simulink model "Dion_CBC_Simulink"  (R2023a)
settings: Solver=ode5  StartTime=0.0  StopTime=Inf  FixedStep=0.001  RelTol=1e-3
PostLoadFcn:
  | , if any(exist('dsrtsu_mdlpostloadfcn', 'file') ~= 0), dsrtsu_mdlpostloadfcn('Execute', bdroot); end,
InitFcn:
  | , if any(exist('rtifpga_mdlclblib', 'file') ~= 0), rtifpga_mdlclblib('Init', bdroot); end,
values from neighbouring files (symbols this model uses):
  k_harmonics = 7    [freq_sweep_continous.m]
libraries: simulink x3, rti1202lib_adc_class1 x3, rti1202lib_dac_class1 x1, rti1202lib_base x1
(part 1 of 2)
Description:
  | Standard RTI1202 template.
  | Supported MATLAB version:  R2023a.
settings Model: Tag=RTI1202  DSRTSU_INTERNAL_RTI_VER=620  DSRTSU_INTERNAL_RTI_TYPE=rti1202  RTICANMMDATA=struct('GeneralSetupData',struct('modelroot','C:\Users\VM-User\Desktop\MigrationScripts','generalsettings',struct('filesettings',struct('destfolder',struct('Name','RTICANMM_FILES','Check',1),'buildfolder',struct('Name','.','Check',1),'AbsDestfolder',struct('Name','C:\Users\VM-User\Desktop\MigrationScripts\RTICANMM_FILES'),'AbsBuildfolder',struct('Name','C:\Users\VM-User\Desktop\MigrationScripts'))),'options',struct('addpaths',1,'rmpaths',1,'addtrcexclusion',true,'cannavigator',struct('checkmonitoring',0),'show_usrtrc',0,'use_usrtrc',0),'advanced',struct('options',ones(1,100)),'MPSetup',{{}},'RTI',struct('Type','RTI1202','Ver','7.17','Date','02-Nov-2021'),'modelname','','block','untitled'))  DSRTSU_INTERNAL_RTIFPGA=200  DSRTSU_INTERNAL_RTISTBM_VER=23.1  Creator=akb110  LastModifiedBy=dionl
settings SolverCC: AlgebraicLoopSolver=TrustRegion
settings DataIOCC: ReturnWorkspaceOutputs=off
settings OptimizationCC: BlockReduction=off  OptimizeBlockIOStorage=off  BufferReuse=off  ReuseModelBlockBuffer=off  GlobalBufferReuse=off  ExpressionFolding=off  LocalBlockOutputs=off  OptimizeDataStoreBuffers=off  BusAssignmentInplaceUpdate=off
settings DebuggingCC: UnconnectedInputMsg=warning  UnconnectedOutputMsg=warning  UnconnectedLineMsg=warning  PregeneratedLibrarySubsystemCodeDiagnostic=none  ArithmeticOperatorsInVariantConditions=warning
settings HardwareCC: ProdBitPerPointer=32  ProdBitPerSizeT=32  ProdBitPerPtrDiffT=32  ProdLargestAtomicInteger=Integer  ProdEndianess=BigEndian  ProdWordSize=32  ProdLongLongMode=on  ProdHWDeviceType=Custom Processor->Custom  TargetIntDivRoundTo=Zero  TargetEndianess=BigEndian  TargetHWDeviceType=Custom Processor->Custom
settings ModelReferenceCC: EnableRefExpFcnMdlSchedulingChecks=on  EnableParallelModelReferenceBuilds=on  ParallelModelReferenceMATLABWorkerInit=Load Top Model
settings SFSimCC: SimUseLocalCustomCode=off  MATLABDynamicMemAlloc=off  CustomCodeUndefinedFunction=UseInterfaceOnly
settings RTWCC: Description=dSPACE DS1202 Hardware Platform  SystemTargetFile=rti1202.tlc  MakeCommand=make_rti  TemplateMakefile=rti1202.tmf  RTWUseLocalCustomCode=off  DLArmComputeVersion=19.05
settings CodeAppCC: StateflowObjectComments=on
settings STFCustomTargetCC: TargetLangStandard=C89/C90 (ANSI)  ParMdlRefBuildCompliant=on  ConcurrentExecutionCompliant=off  GRTInterface=off  UseToolchainInfoCompliant=off  SystemTargetFile=rti1202.tlc
settings GRTTargetCC: TargetLangStandard=C89/C90 (ANSI)  CompOptLevelCompliant=off  ConcurrentExecutionCompliant=off  CombineOutputUpdateFcns=off  MatFileLogging=off  CPPClassGenCompliant=off  UseToolchainInfoCompliant=off
settings ConfigComp: CovMetricSettings=dswe

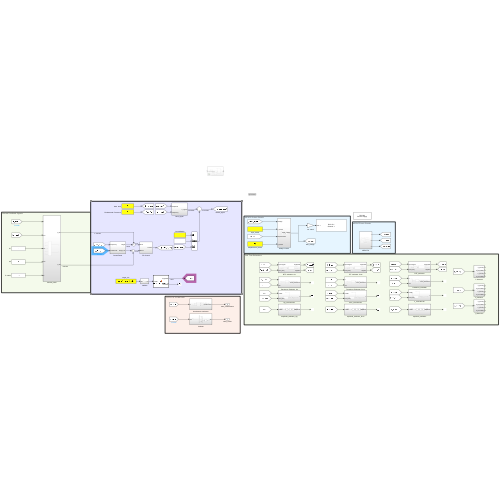
[thumbnail: Simulink's stored preview of the top-level diagram]
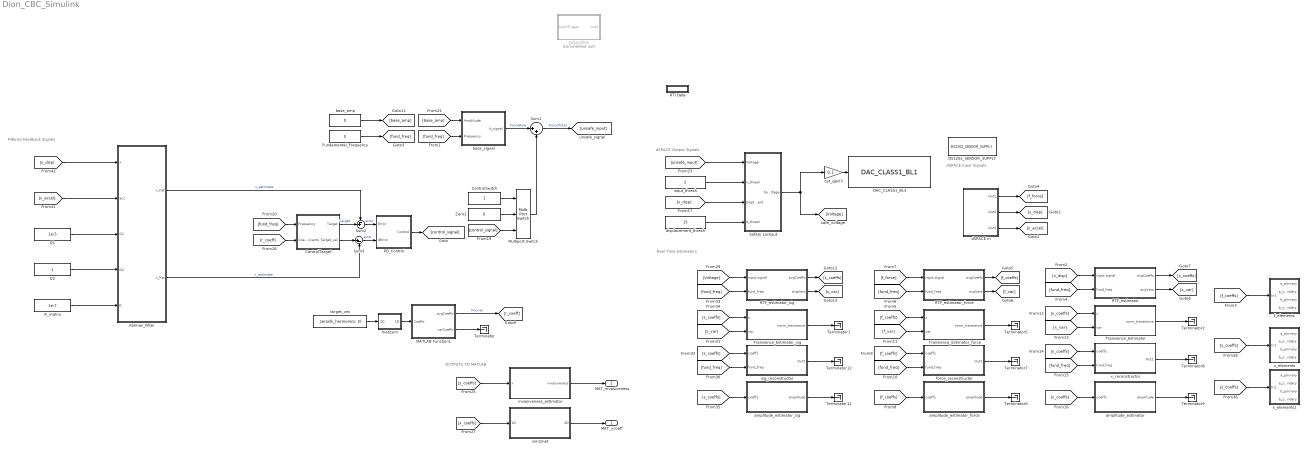
== system Dion_CBC_Simulink ==
  note: OUTPUTS TO MATLAB
  note: Filtered Feedback Signals
  note: Real Time Estimators
  note: dSPACE Input Signals
  note: dSPACE Output Signals
  ControlSwitch : Constant
  ControlTarget : Subsystem
  DAC_CLASS1_BL3 : rti1202lib_dac_class1/DAC_CLASS1_BL1  DSProperties=struct('RTI',struct('Version',uint32(2),'BlockType',struct('isSLSource',uint8(0),'isSLSink',uint8(1),'isHWSource',uint8(0),'isHWSink',uint8(1),'isSetup',uint8(0),'isInline',uint8(1),'isNonInline',uint8(0),'isInterrupt',uint8(0),'isChannelwise',uint8(1)),'IOBoardType',{{'DS120X','STD','DACC1'}},'UnitType','DAC','Identifier','DAC','DialogType','ML','BlockSet','NONE','SlaveProcessor','NONE'))  RTIBlockInterface=struct('InputPortsActive',1,'InputPortsWidth',int32(1),'InputPortsDataType',{{'SS_DOUBLE'}},'InputPortsName',{{['DAC 1']}},'DialogFcn','rti120xstddacc1dacgui','InitLevel',3,'IconTransparency','on','BlockDisplay',{{['DAC CL1\nChannel: 1'],'center'}},'BlockName',struct('Token',{{'DAC_CLASS1_BL1'}}))  RTIBlockParameters=struct('ChannelNo',{{1,'OFF',[]}},'ChannelNumOf',{{1,'OFF',[]}},'InitialValue1',{{0,'OFF',[-10 10]}},'InitialValue2',{{0,'OFF',[-10 10]}},'InitialValue3',{{0,'OFF',[-10 10]}},'InitialValue4',{{0,'OFF',[-10 10]}},'InitialValue5',{{0,'OFF',[-10 10]}},'InitialValue6',{{0,'OFF',[-10 10]}},'InitialValue7',{{0,'OFF',[-10 10]}},'InitialValue8',{{0,'OFF',[-10 10]}},'InitialValue9',{{0,'OFF',[-10 10]}},'InitialValue10',{{0,'OFF',[-10 10]}},'InitialValue11',{{0,'OFF',[-10 10]}},'InitialValue12',{{0,'OFF',[-10 10]}},'InitialValue13',{{0,'OFF',[-10 10]}},'InitialValue14',{{0,'OFF',[-10 10]}},'InitialValue15',{{0,'OFF',[-10 10]}},'InitialValue16',{{0,'OFF',[-10 10]}},'OutputMode',{{ones(1,16),'OFF',[1 2]}},'TermValue1',{{0,'OFF',[-10 10]}},'TermValue2',{{0,'OFF',[-10 10]}},'TermValue3',{{0,'OFF',[-10 10]}},'TermValue4',{{0,'OFF',[-10 10]}},'TermValue5',{{0,'OFF',[-10 10]}},'TermValue6',{{0,'OFF',[-10 10]}},'TermValue7',{{0,'OFF',[-10 10]}},'TermValue8',{{0,'OFF',[-10 10]}},'TermValue9',{{0,'OFF',[-10 10]}},'TermValue10',{{0,'OFF',[-10 10]}},'TermValue11',{{0,'OFF',[-10 10]}},'TermValue12',{{0,'OFF',[-10 10]}},'TermValue13',{{0,'OFF',[-10 10]}},'TermValue14',{{0,'OFF',[-10 10]}},'TermValue15',{{0,'OFF',[-10 10]}},'TermValue16',{{0,'OFF',[-10 10]}},'EnableTermMode',{{0,'OFF',[0 1]}},'TLCFileName',{{'rti120xdac_c1_dac','OFF',[]}},'InitialValueBuildCheck1',{{0,'OFF',[]}},'InitialValueBuildCheck2',{{0,'OFF',[]}},'InitialValueBuildCheck3',{{0,'OFF',[]}},'InitialValueBuildCheck4',{{0,'OFF',[]}},'InitialValueBuildCheck5',{{0,'OFF',[]}},'InitialValueBuildCheck6',{{0,'OFF',[]}},'InitialValueBuildCheck7',{{0,'OFF',[]}},'InitialValueBuildCheck8',{{0,'OFF',[]}},'InitialValueBuildCheck9',{{0,'OFF',[]}},'InitialValueBuildCheck10',{{0,'OFF',[]}},'InitialValueBuildCheck11',{{0,'OFF',[]}},'InitialValueBuildCheck12',{{0,'OFF',[]}},'InitialValueBuildCheck13',{{0,'OFF',[]}},'InitialValueBuildCheck14',{{0,'OFF',[]}},'InitialValueBuildCheck15',{{0,'OFF',[]}},'InitialValueBuildCheck16',{{0,'OFF',[]}},'TermValueBuildCheck1',{{0,'OFF',[]}},'TermValueBuildCheck2',{{0,'OFF',[]}},'TermValueBuildCheck3',{{0,'OFF',[]}},'TermValueBuildCheck4',{{0,'OFF',[]}},'TermValueBuildCheck5',{{0,'OFF',[]}},'TermValueBuildCheck6',{{0,'OFF',[]}},'TermValueBuildCheck7',{{0,'OFF',[]}},'TermValueBuildCheck8',{{0,'OFF',[]}},'TermValueBuildCheck9',{{0,'OFF',[]}},'TermValueBuildCheck10',{{0,'OFF',[]}},'TermValueBuildCheck11',{{0,'OFF',[]}},'TermValueBuildCheck12',{{0,'OFF',[]}},'TermValueBuildCheck13',{{0,'OFF',[]}},'TermValueBuildCheck14',{{0,'OFF',[]}},'TermValueBuildCheck15',{{0,'OFF',[]}},'TermValueBuildCheck16',{{0,'OFF',[]}})  RTISFcnParameters=struct('ChannelNo','int16','ChannelNumOf','int16','InitialValue1','double','InitialValue2','double','InitialValue3','double','InitialValue4','double','InitialValue5','double','InitialValue6','double','InitialValue7','double','InitialValue8','double','InitialValue9','double','InitialValue10','double','InitialValue11','double','InitialValue12','double','InitialValue13','double','InitialValue14','double','InitialValue15','double','InitialValue16','double','OutputMode','int16','TermValue1','double','TermValue2','double','TermValue3','double','TermValue4','double','TermValue5','double','TermValue6','double','TermValue7','double','TermValue8','double','TermValue9','double','TermValue10','double','TermValue11','double','TermValue12','double','TermValue13','double','TermValue14','double','TermValue15','double','TermValue16','double','EnableTermMode','int16','TLCFileName','char')  RTIBlockParaDefault=struct('ChannelNo',1,'ChannelNumOf',1,'InitialValue1',0,'InitialValue2',0,'InitialValue3',0,'InitialValue4',0,'InitialValue5',0,'InitialValue6',0,'InitialValue7',0,'InitialValue8',0,'InitialValue9',0,'InitialValue10',0,'InitialValue11',0,'InitialValue12',0,'InitialValue13',0,'InitialValue14',0,'InitialValue15',0,'InitialValue16',0,'OutputMode',ones(1,16),'TermValue1',0,'TermValue2',0,'TermValue3',0,'TermValue4',0,'TermValue5',0,'TermValue6',0,'TermValue7',0,'TermValue8',0,'TermValue9',0,'TermValue10',0,'TermValue11',0,'TermValue12',0,'TermValue13',0,'TermValue14',0,'TermValue15',0,'TermValue16',0,'EnableTermMode',0,'TLCFileName','rti120xdac_c1_dac','InitialValueBuildCheck1',0,'InitialValueBuildCheck2',0,'InitialValueBuildCheck3',0,'InitialValueBuildCheck4',0,'InitialValueBuildCheck5',0,'InitialValueBuildCheck6',0,'InitialValueBuildCheck7',0,'InitialValueBuildCheck8',0,'InitialValueBuildCheck9',0,'InitialValueBuildCheck10',0,'InitialValueBuildCheck11',0,'InitialValueBuildCheck12',0,'InitialValueBuildCheck13',0,'InitialValueBuildCheck14',0,'InitialValueBuildCheck15',0,'InitialValueBuildCheck16',0,'TermValueBuildCheck1',0,'TermValueBuildCheck2',0,'TermValueBuildCheck3',0,'TermValueBuildCheck4',0,'TermValueBuildCheck5',0,'TermValueBuildCheck6',0,'TermValueBuildCheck7',0,'TermValueBuildCheck8',0,'TermValueBuildCheck9',0,'TermValueBuildCheck10',0,'TermValueBuildCheck11',0,'TermValueBuildCheck12',0,'TermValueBuildCheck13',0,'TermValueBuildCheck14',0,'TermValueBuildCheck15',0,'TermValueBuildCheck16',0)
  DS1202_SENSOR_SUPPLY : rti1202lib_base/DS1202_SENSOR_SUPPLY  DSProperties=struct('RTI',struct('Version',uint32(1),'BlockType',struct('isSLSource',uint8(0),'isSLSink',uint8(0),'isHWSource',uint8(0),'isHWSink',uint8(1),'isSetup',uint8(0),'isInline',uint8(1),'isNonInline',uint8(0),'isInterrupt',uint8(0),'isChannelwise',uint8(0)),'IOBoardType',{{'DS120X','BASE'}},'UnitType','SENSORSUPPLY','Identifier','SENSORSUPPLY','DialogType','ML','BlockSet','NONE','SlaveProcessor','NONE'))  RTIBlockInterface=struct('OutputPortsActive',0,'OutputPortsWidth',int32(0),'DialogFcn','rti120xbasesensorsupplygui','InitLevel',3,'IconTransparency','off','BlockDisplay',{{['DS1202\nSensor Supply'],'center'}},'BlockName',struct('Token',{{'DS1202_SENSOR_SUPPLY'}}))  RTIBlockParameters=struct('Voltage',{{'14','OFF',[2 20]}},'TLCFileName',{{'rti120xbase_sensor_supply','OFF',[]}})  RTISFcnParameters=struct('Voltage','double','TLCFileName','char')  RTIBlockParaDefault=struct('Voltage',2,'TLCFileName','rti120xbase_sensor_supply')
  Fundamental_Frequency : Constant  Value=5
  Kalman_Filter : Subsystem
  MATLAB Function1 : MATLAB Function  TreatAsAtomicUnit=on
  Multiport Switch : MultiPortSwitch  Inputs=2  SaturateOnIntegerOverflow=off  InputSameDT=off
  PD_Control : Subsystem
  Q1 : Constant  Value=1e-5
  Q2 : Constant
  RTF_estimator : Subsystem
  RTF_estimator_force : Subsystem
  RTF_estimator_sig : Subsystem
  RTI Data : Subsystem  Tag=struct('RTIDataServer',struct('RTIDataServerVs','2','RTIModelDescription','struct(''main'',''Dion_CBC_Simulink'',''sub'',''Dion_CBC_Simulink'',''isMp'',0)'))  LoadFcn="if exist('rtidc'), try,  rtidc('DataHostBlockClbLoad', gcbh); catch, disp(['Warning: ''LoadFcn'' for RTI Data block failed: ' lasterr]); end, end,"  mask(RTI_DATA_HOST){}
      mask help:
      | RTI Data Block.
      | This block is used by RTI to store internal model-dependent data.
      | Please keep this block on the root level of the model. Deleting this block will result in data loss.
      |
      | NEVER DELETE OR COPY THIS BLOCK!
      settings: CopyFcn="if exist('rtidc'), try,  rtidc('DataHostBlockClbCopy', gcbh); catch, disp(['Warning: ''CopyFcn'' for RTI Data block failed: ' lasterr]); end, end,"  DeleteFcn="if exist('rtidc'), try,  rtidc('DataHostBlockClbDelete', gcbh); catch, disp(['Warning: ''DeleteFcn'' for RTI Data block failed: ' lasterr]); end, end,"  ModelCloseFcn="if exist('rtidc'), try,  rtidc('DataHostBlockClbModelClose', gcbh); catch, disp(['Warning: ''ModelCloseFcn'' for RTI Data block failed: ' lasterr]); end, end,"  PreSaveFcn="if exist('rtidc'), try,  rtidc('DataHostBlockClbPreSave', gcbh); catch, disp(['Warning: ''PreSaveFcn'' for RTI Data block failed: ' lasterr]); end, end,"  PostSaveFcn="if exist('rtidc'), try,  rtidc('DataHostBlockClbPostSave', gcbh); catch, disp(['Warning: ''PostSaveFcn'' for RTI Data block failed: ' lasterr]); end, end,"  NameChangeFcn="if exist('rtidc'), try,  rtidc('DataHostBlockClbNameChange', gcbh); catch, disp(['Warning: ''NameChangeFcn'' for RTI Data block failed: ' lasterr]); end, end,"
      mask Help:
      | RTI Data Block.
      | This block is used by RTI to store internal model-dependent data.
      | Please keep this block on the root level of the model. Deleting this block will result in data loss.
      | 
      | NEVER DELETE OR COPY THIS BLOCK!
      mask Display:
      | text(0.5, 0.5, 'RTI Data', 'HorizontalAlignment', 'center');
      | plot([1 0]);
  R_matrix : Constant  Value=1e-7
  Safety Lockout : Subsystem
  Subsystem : Subsystem  Commented=on
  Sum1 : Sum  Inputs=|++
  Sum2 : Sum  Inputs=-+|
  Sum3 : Sum  Inputs=|+-
  Terminator{,1..2,5..9,11..12} (10 alike) : Terminator
  Transience_Estimator : Subsystem
  Transience_Estimator_force : Subsystem
  Transience_Estimator_sig : Subsystem
  Zero2 : Constant  Value=0
  amplitude_estimator : Subsystem
  amplitude_estimator_force : Subsystem
  amplitude_estimator_sig : Subsystem
  base_amp : Constant  Value=0
  base_signal : Subsystem
  dSPACE in : Subsystem
  displacement_thresh : Constant  Value=15
  f_elements : Subsystem
  force_reconstructor : Subsystem
  input_thresh : Constant  Value=2
  invasiveness_estimator : Subsystem
  mat2sim : Subsystem
  out_gain3 : Gain  Gain=0.1
  sig_reconstructor : Subsystem
  sim2mat : Subsystem
  target_vec : Constant  Value=zeros(k_harmonics, 2)
  x_elements : Subsystem
  x_elements1 : Subsystem
  x_reconstructor : Subsystem
  MAT_xcoeff : Outport
  MAT_invasiveness : Outport  Port=2
  wires:
  dSPACE in/3(Out3) -> [x_accel]
  [x_disp] -> RTF_estimator/1(input signal)
  [fund_freq] -> RTF_estimator/2(fund_freq)
  Fundamental_Frequency/1 -> [fund_freq]
  amplitude_estimator_force/1(amplitude) -> Terminator6/1
  Transience_Estimator_force/1(norm_transience) -> Terminator5/1
  [fund_freq] -> RTF_estimator_force/2(fund_freq)
  [f_force] -> RTF_estimator_force/1(input signal)
  force_reconstructor/1(Out1) -> Terminator7/1
  RTF_estimator_force/1(avgCoeffs) -> [f_coeffs]
  [f_coeffs] -> Transience_Estimator_force/1(x)
  [f_coeffs] -> amplitude_estimator_force/1(coeffs)
  [f_coeffs] -> force_reconstructor/1(coeffs)
  [fund_freq] -> force_reconstructor/2(fund_freq)
  RTF_estimator_force/2(avgVars) -> [f_var]
  [f_var] -> Transience_Estimator_force/2(var)
  RTF_estimator/1(avgCoeffs) -> [x_coeffs]
  RTF_estimator/2(avgVars) -> [x_var]
  [x_coeffs] -> Transience_Estimator/1(x)
  [x_var] -> Transience_Estimator/2(var)
  Transience_Estimator/1(norm_transience) -> Terminator2/1
  [x_coeffs] -> x_reconstructor/1(coeffs)
  [fund_freq] -> x_reconstructor/2(fund_freq)
  [x_coeffs] -> amplitude_estimator/1(coeffs)
  amplitude_estimator/1(amplitude) -> Terminator9/1
  x_reconstructor/1(Out1) -> Terminator8/1
  [fund_freq] -> base_signal/2(Frequency)
  base_signal/1(b_signal) -> Sum1/1  "ForceRaw"
  Sum1/1 -> [unsafe_input]  "ForceTotal"
  ControlSwitch/1 -> Multiport Switch/1
  Zero2/1 -> Multiport Switch/2
  [control_signal] -> Multiport Switch/3
  Sum2/1 -> PD_Control/1(Error)  "error"
  PD_Control/1(Control) -> [control_signal]
  [fund_freq] -> ControlTarget/1(Frequency)
  Multiport Switch/1 -> Sum1/2
  [x_coeffs] -> sim2mat/1(1D)
  [base_amp] -> base_signal/1(Amplitude)
  [r_coeff] -> ControlTarget/2(Coefficients)
  dSPACE in/2(Out2) -> [x_disp]
  dSPACE in/1(Out1) -> [f_force]
  base_amp/1 -> [base_amp]
  [f_coeffs] -> f_elements/1(In1)
  [x_coeffs] -> x_elements/1(In1)
  [s_coeffs] -> invasiveness_estimator/1(x)
  invasiveness_estimator/1(invasiveness) -> MAT_invasiveness/1
  [s_var] -> Transience_Estimator_sig/2(var)
  RTF_estimator_sig/2(avgVars) -> [s_var]
  [fund_freq] -> sig_reconstructor/2(fund_freq)
  [s_coeffs] -> sig_reconstructor/1(coeffs)
  [s_coeffs] -> amplitude_estimator_sig/1(coeffs)
  [s_coeffs] -> Transience_Estimator_sig/1(x)
  RTF_estimator_sig/1(avgCoeffs) -> [s_coeffs]
  sig_reconstructor/1(Out1) -> Terminator12/1
  [Voltage] -> RTF_estimator_sig/1(input signal)
  [fund_freq] -> RTF_estimator_sig/2(fund_freq)
  Transience_Estimator_sig/1(norm_transience) -> Terminator1/1
  amplitude_estimator_sig/1(amplitude) -> Terminator11/1
  [s_coeffs] -> x_elements1/1(In1)
  Q2/1 -> Kalman_Filter/4(Q2)
  R_matrix/1 -> Kalman_Filter/5(R)
  Kalman_Filter/2(v_hat) -> Sum3/2  "v_estimate"
  Kalman_Filter/1(x_hat) -> Sum2/1  "x_estimate"
  [x_disp] -> Kalman_Filter/1(x)
  [x_accel] -> Kalman_Filter/2(acc)
  Q1/1 -> Kalman_Filter/3(Q1)
  ControlTarget/1(Target) -> Sum2/2  "Target"
  ControlTarget/2(Target_vel) -> Sum3/1
  Sum3/1 -> PD_Control/2(dError)  "error"
  MATLAB Function1/1(avgCoeffs) -> [r_coeff]  "Fourier"
  target_vec/1 -> mat2sim/1(2D)
  MATLAB Function1/2(varCoeffs) -> Terminator/1
  mat2sim/1(1D) -> MATLAB Function1/1(Coeffs)
  sim2mat/1(2D) -> MAT_xcoeff/1
  [unsafe_input] -> Safety Lockout/1(Voltage)
  input_thresh/1 -> Safety Lockout/2(v_thresh)
  [x_disp] -> Safety Lockout/3(Displacement)
  displacement_thresh/1 -> Safety Lockout/4(d_thresh)
  Safety Lockout/1(Safe_Voltage) -> out_gain3/1, [Voltage]
  out_gain3/1 -> DAC_CLASS1_BL3/1

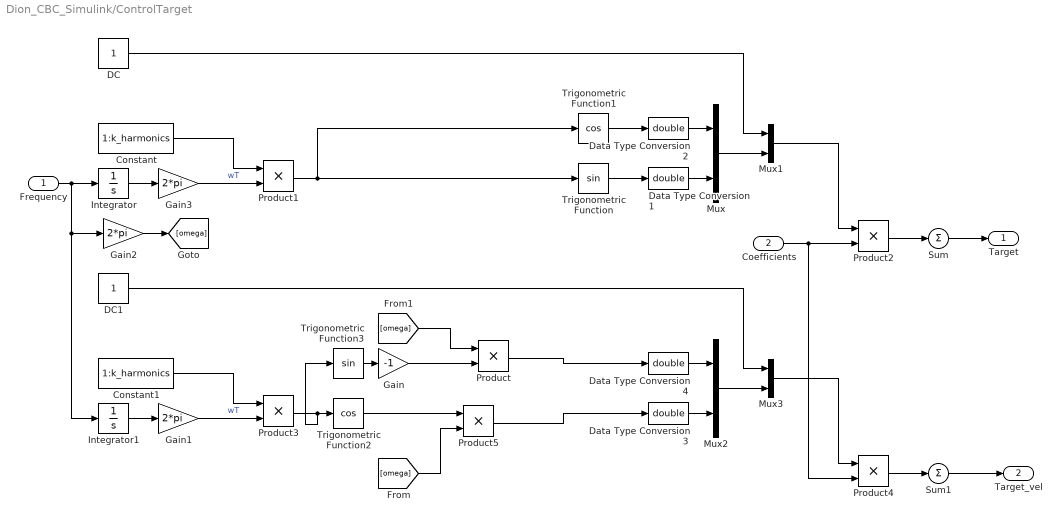
== system Dion_CBC_Simulink/ControlTarget ==
  Frequency : Inport
  Coefficients : Inport  Port=2
  Constant : Constant  Value=1:k_harmonics
  Constant1 : Constant  Value=1:k_harmonics
  DC : Constant
  DC1 : Constant
  Data Type Conversion{1..4} (4 alike) : DataTypeConversion  OutDataTypeStr=double  SaturateOnIntegerOverflow=off  RndMeth=Floor
  Gain : Gain  Gain=-1
  Gain1 : Gain  Gain=2*pi
  Gain2 : Gain  Gain=2*pi
  Gain3 : Gain  Gain=2*pi
  Integrator : Integrator
  Integrator1 : Integrator
  Mux{,1..3} (4 alike) : Mux  Inputs=2
  Product{,1,3,5} (4 alike) : Product
  Product2 : Product  RndMeth=Zero
  Product4 : Product  RndMeth=Zero
  Sum : Sum  Inputs=|+|
  Sum1 : Sum  Inputs=|+|
  Trigonometric Function : Trigonometry
  Trigonometric Function1 : Trigonometry  Operator=cos
  Trigonometric Function2 : Trigonometry  Operator=cos
  Trigonometric Function3 : Trigonometry
  Target : Outport
  Target_vel : Outport  Port=2
  wires:
  Product2/1 -> Sum/1
  Product1/1 -> Trigonometric Function1/1, Trigonometric Function/1
  Sum/1 -> Target/1
  Integrator/1 -> Gain3/1
  Constant/1 -> Product1/1
  Trigonometric Function/1 -> Data Type Conversion1/1
  Mux1/1 -> Product2/1
  Trigonometric Function1/1 -> Data Type Conversion2/1
  Data Type Conversion2/1 -> Mux/1
  Data Type Conversion1/1 -> Mux/2
  Mux/1 -> Mux1/2
  DC/1 -> Mux1/1
  Gain3/1 -> Product1/2  "wT"
  Gain1/1 -> Product3/2  "wT"
  DC1/1 -> Mux3/1
  Mux2/1 -> Mux3/2
  Data Type Conversion3/1 -> Mux2/2
  Data Type Conversion4/1 -> Mux2/1
  Coefficients/1 -> Product4/2, Product2/2
  Trigonometric Function3/1 -> Gain/1
  Mux3/1 -> Product4/1
  Trigonometric Function2/1 -> Product5/1
  Constant1/1 -> Product3/1
  Integrator1/1 -> Gain1/1
  Frequency/1 -> Integrator1/1, Gain2/1, Integrator/1
  Sum1/1 -> Target_vel/1
  Product3/1 -> Trigonometric Function2/1, Trigonometric Function3/1
  Product4/1 -> Sum1/1
  Gain2/1 -> [omega]
  [omega] -> Product/1
  [omega] -> Product5/2
  Product/1 -> Data Type Conversion4/1
  Gain/1 -> Product/2
  Product5/1 -> Data Type Conversion3/1

== system Dion_CBC_Simulink/Kalman_Filter ==
  x : Inport
  acc : Inport  Port=2
  Q1 : Inport  Port=3
  Q2 : Inport  Port=4
  R : Inport  Port=5
  MATLAB Function : MATLAB Function  TreatAsAtomicUnit=on
  x_hat : Outport
  v_hat : Outport  Port=2
  wires:
  R/1 -> MATLAB Function/5(R)
  Q1/1 -> MATLAB Function/3(q1)
  Q2/1 -> MATLAB Function/4(q2)
  acc/1 -> MATLAB Function/2(acc_measured)
  x/1 -> MATLAB Function/1(disp_measured)
  MATLAB Function/1(disp_estimate) -> x_hat/1
  MATLAB Function/2(vel_estimate) -> v_hat/1

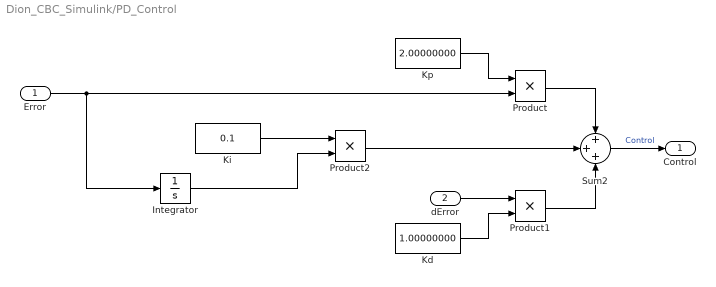
== system Dion_CBC_Simulink/PD_Control ==
  Error : Inport
  dError : Inport  Port=2
  Integrator : Integrator
  Kd : Constant  Value=1.00000000
  Ki : Constant  Value=0.1
  Kp : Constant  Value=2.00000000
  Product : Product  RndMeth=Zero
  Product1 : Product  RndMeth=Zero
  Product2 : Product  RndMeth=Zero
  Sum2 : Sum  Inputs=+++
  Control : Outport
  wires:
  Kp/1 -> Product/1
  Kd/1 -> Product1/2
  Product/1 -> Sum2/1
  Product1/1 -> Sum2/3
  Error/1 -> Integrator/1, Product/2
  Sum2/1 -> Control/1  "Control"
  dError/1 -> Product1/1
  Ki/1 -> Product2/1
  Product2/1 -> Sum2/2
  Integrator/1 -> Product2/2

== system Dion_CBC_Simulink/RTF_estimator ==
  input signal : Inport
  fund_freq : Inport  Port=2
  MATLAB Function1 : MATLAB Function  TreatAsAtomicUnit=on
  Subsystem : Subsystem
  Terminator : Terminator
  avgCoeffs : Outport
  avgVars : Outport  Port=2
  wires:
  input signal/1 -> Subsystem/1(input signal)
  Subsystem/2(Phase1) -> Terminator/1
  fund_freq/1 -> Subsystem/2(fund_freq)
  Subsystem/1(Fourier1) -> MATLAB Function1/1(Coeffs)
  MATLAB Function1/2(varCoeffs) -> avgVars/1
  MATLAB Function1/1(avgCoeffs) -> avgCoeffs/1  "Fourier"

== system Dion_CBC_Simulink/RTF_estimator_force ==
  input signal : Inport
  fund_freq : Inport  Port=2
  MATLAB Function1 : MATLAB Function  TreatAsAtomicUnit=on
  Subsystem : Subsystem
  Terminator : Terminator
  avgCoeffs : Outport
  avgVars : Outport  Port=2
  wires:
  MATLAB Function1/1(avgCoeffs) -> avgCoeffs/1  "Fourier"
  MATLAB Function1/2(varCoeffs) -> avgVars/1
  Subsystem/1(Fourier1) -> MATLAB Function1/1(Coeffs)
  fund_freq/1 -> Subsystem/2(fund_freq)
  Subsystem/2(Phase1) -> Terminator/1
  input signal/1 -> Subsystem/1(input signal)

== system Dion_CBC_Simulink/RTF_estimator_sig ==
  input signal : Inport
  fund_freq : Inport  Port=2
  MATLAB Function1 : MATLAB Function  TreatAsAtomicUnit=on
  Subsystem : Subsystem
  Terminator : Terminator
  avgCoeffs : Outport
  avgVars : Outport  Port=2
  wires:
  input signal/1 -> Subsystem/1(input signal)
  Subsystem/2(Phase1) -> Terminator/1
  fund_freq/1 -> Subsystem/2(fund_freq)
  Subsystem/1(Fourier1) -> MATLAB Function1/1(Coeffs)
  MATLAB Function1/2(varCoeffs) -> avgVars/1
  MATLAB Function1/1(avgCoeffs) -> avgCoeffs/1  "Fourier"

== system Dion_CBC_Simulink/RTI Data ==
  RTI Data Store : Subsystem  Tag="struct('public',struct('sub',struct('name',{{'Dion_CBC_Simulink'}},'data',{{struct('TH',struct('thTaskInfo',struct('taskType',{'TIMER','HWINT','TMRINT','SWINT','GLINT'},'tasksNumOf',{1,0,0,0,0},'srcIds',{{'TIMERA'},{},{},{},{}},'taskNames',{{['Timer Task 1']},{},{},{},{}})),'th_tc',struct('dataType','TASK','taskGroupId','','taskGroupList',{{}},'taskSchedulingPolicy','FCFS','taskType','TIMER','blkh',-1,'srcId','TIMERA','srcSgnName',['Timer A interrupt'],'srcCpuName','','taskName',['Timer Task 1  [0.001] s'],'taskNameDisplayExt','','smplTime',0.001,'smplTimeOffs',0,'hasFixedPriority',0,'priority',1,'hasFixedOvc',0,'ovcType',1,'ovcMax',1),'tc_th',struct('dataType','TASK','taskGroupId','','taskGroupList',{{}},'taskSchedulingPolicy','FCFS','taskType','TIMER','blkh',-1,'srcId','TIMERA','srcSgnName',['Timer A interrupt'],'srcCpuName','','taskName',['Timer Task 1  [0.001] s'],'taskNameDisplayExt','','smplTime',0.001,'smplTimeOffs',0,'hasFixedPriority',0,'priority',1,'hasFixedOvc',0,'ovcType',1,'ovcMax',1))}})),'private',struct('version',struct('dsVer',uint32(2)),'access',struct('modified',['01-Aug-2025 12:46:06'],'type','Model','isPerm',1)))"  mask(RTI_DATA_STORE){}
      mask help:
      | RTI Data Store Block. This block is used by RTI to store internal model dependent data. Deleting this block will result in data loss.
      |
      | NEVER DELETE, COPY, OR MODIFY THIS BLOCK!
      mask Help:
      | RTI Data Store Block. This block is used by RTI to store internal model dependent data. Deleting this block will result in data loss.
      | 
      | NEVER DELETE, COPY, OR MODIFY THIS BLOCK!
      mask Display: text(0.5, 0.5, ' ', 'HorizontalAlignment', 'center');

== system Dion_CBC_Simulink/Safety Lockout ==
  Voltage : Inport
  v_thresh : Inport  Port=2
  Displacement : Inport  Port=3
  d_thresh : Inport  Port=4
  AND : Logic  IconShape=distinctive  AllPortsSameDT=off  OutDataTypeStr=boolean
  No_input1 : Constant  Value=0
  amplitude_switch : Switch  Criteria=u2 > Threshold  SaturateOnIntegerOverflow=off  InputSameDT=off
  input_safety : Subsystem
  output_safety : Subsystem
  Safe_Voltage : Outport
  wires:
  output_safety/1(valid) -> AND/2
  d_thresh/1 -> output_safety/2(threshold)
  input_safety/1(valid) -> AND/1
  amplitude_switch/1 -> Safe_Voltage/1
  No_input1/1 -> amplitude_switch/3
  Voltage/1 -> amplitude_switch/1, input_safety/1(signal)
  v_thresh/1 -> input_safety/2(threshold)
  AND/1 -> amplitude_switch/2
  Displacement/1 -> output_safety/1(signal)

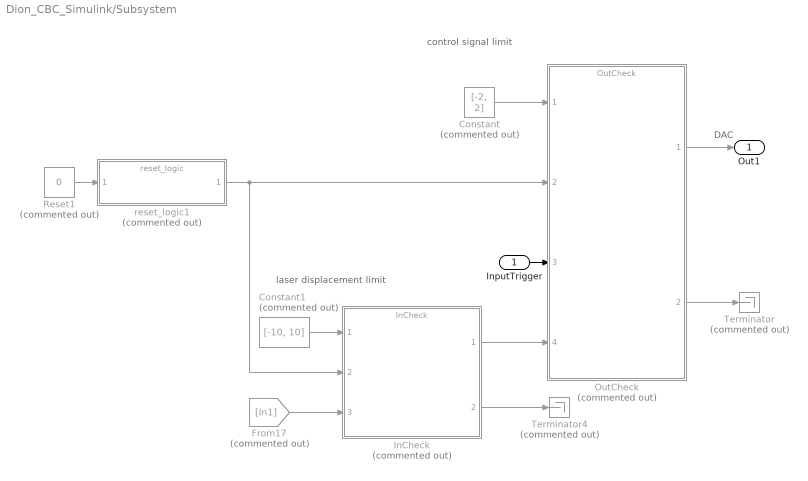
== system Dion_CBC_Simulink/Subsystem ==
  note: DAC
  note: control signal limit
  note: laser displacement limit
  InputTrigger : Inport
  Constant : Constant  Commented=on  Value=[-2, 2]
  Constant1 : Constant  Commented=on  Value=[-10, 10]
  From17 : From  Commented=on  GotoTag=In1
  InCheck : ModelReference  Commented=on  ModelNameDialog=InCheck.slxp  ModelReferenceVersion=1.2  CopyOfModelProtected=on
  OutCheck : ModelReference  Commented=on  ModelNameDialog=OutCheck.slxp  ModelReferenceVersion=1.2  CopyOfModelProtected=on
  Reset1 : Constant  Commented=on  Value=0
  Terminator : Terminator  Commented=on
  Terminator4 : Terminator  Commented=on
  reset_logic1 : ModelReference  Commented=on  ModelNameDialog=reset_logic.slxp  ModelReferenceVersion=1.2  CopyOfModelProtected=on
  Out1 : Outport
  wires:
  InCheck/1 -> OutCheck/4
  InputTrigger/1 -> OutCheck/3
  Reset1/1 -> reset_logic1/1
  OutCheck/2 -> Terminator/1
  reset_logic1/1 -> OutCheck/2, InCheck/2
  From17/1 -> InCheck/3
  InCheck/2 -> Terminator4/1
  OutCheck/1 -> Out1/1
  Constant/1 -> OutCheck/1
  Constant1/1 -> InCheck/1

== system Dion_CBC_Simulink/Transience_Estimator ==
  x : Inport
  var : Inport  Port=2
  Abs1 : Abs  SaturateOnIntegerOverflow=off
  Divide2 : Product  Inputs=*/
  Max : MinMax  Function=max
  get primary1 : Subsystem
  get primary4 : Subsystem
  norm_transience : Outport
  wires:
  Divide2/1 -> Abs1/1
  x/1 -> get primary1/1(Vector)
  get primary1/1(Primary) -> Divide2/2
  get primary4/1(Primary) -> Divide2/1
  var/1 -> get primary4/1(Vector)
  Abs1/1 -> Max/1
  Max/1 -> norm_transience/1

== system Dion_CBC_Simulink/Transience_Estimator_force ==
  x : Inport
  var : Inport  Port=2
  Abs1 : Abs  SaturateOnIntegerOverflow=off
  Divide2 : Product  Inputs=*/
  Max : MinMax  Function=max
  get primary1 : Subsystem
  get primary4 : Subsystem
  norm_transience : Outport
  wires:
  Max/1 -> norm_transience/1
  Abs1/1 -> Max/1
  var/1 -> get primary4/1(Vector)
  get primary4/1(Primary) -> Divide2/1
  get primary1/1(Primary) -> Divide2/2
  x/1 -> get primary1/1(Vector)
  Divide2/1 -> Abs1/1

== system Dion_CBC_Simulink/Transience_Estimator_sig ==
  x : Inport
  var : Inport  Port=2
  Abs1 : Abs  SaturateOnIntegerOverflow=off
  Divide2 : Product  Inputs=*/
  Max : MinMax  Function=max
  get primary1 : Subsystem
  get primary4 : Subsystem
  norm_transience : Outport
  wires:
  Divide2/1 -> Abs1/1
  x/1 -> get primary1/1(Vector)
  get primary1/1(Primary) -> Divide2/2
  get primary4/1(Primary) -> Divide2/1
  var/1 -> get primary4/1(Vector)
  Abs1/1 -> Max/1
  Max/1 -> norm_transience/1

== system Dion_CBC_Simulink/amplitude_estimator ==
  coeffs : Inport
  Sqrt : Sqrt
  Square : Math  Operator=square
  Sum of Elements : Sum  Inputs=+
  amplitude : Outport
  wires:
  Sum of Elements/1 -> Sqrt/1
  Square/1 -> Sum of Elements/1
  coeffs/1 -> Square/1
  Sqrt/1 -> amplitude/1

== system Dion_CBC_Simulink/amplitude_estimator_force ==
  coeffs : Inport
  Sqrt : Sqrt
  Square : Math  Operator=square
  Sum of Elements : Sum  Inputs=+
  amplitude : Outport
  wires:
  Sqrt/1 -> amplitude/1
  coeffs/1 -> Square/1
  Square/1 -> Sum of Elements/1
  Sum of Elements/1 -> Sqrt/1

== system Dion_CBC_Simulink/amplitude_estimator_sig ==
  coeffs : Inport
  Sqrt : Sqrt
  Square : Math  Operator=square
  Sum of Elements : Sum  Inputs=+
  amplitude : Outport
  wires:
  Sum of Elements/1 -> Sqrt/1
  Square/1 -> Sum of Elements/1
  coeffs/1 -> Square/1
  Sqrt/1 -> amplitude/1

== system Dion_CBC_Simulink/base_signal ==
  Amplitude : Inport
  Frequency : Inport  Port=2
  Gain : Gain  Gain=2*pi
  Integrator : Integrator
  Product : Product
  Sin : Trigonometry
  b_signal : Outport
  wires:
  Frequency/1 -> Integrator/1
  Gain/1 -> Sin/1
  Amplitude/1 -> Product/1
  Integrator/1 -> Gain/1
  Sin/1 -> Product/2
  Product/1 -> b_signal/1

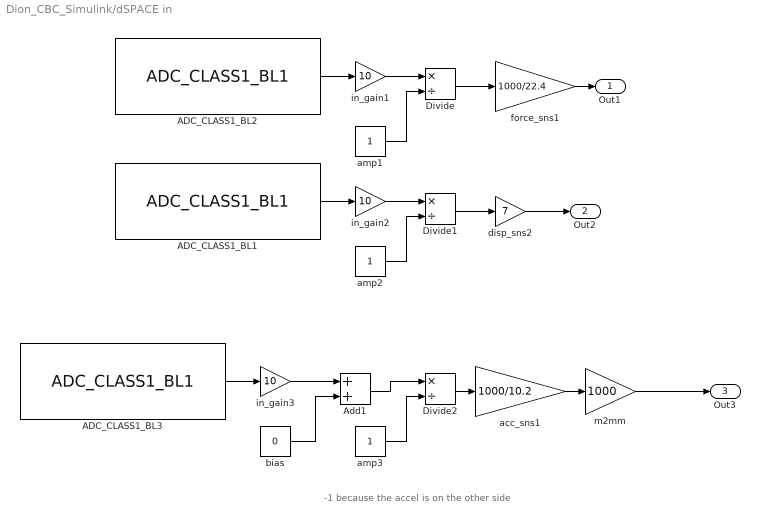
== system Dion_CBC_Simulink/dSPACE in ==
  note: -1 because the accel is on the other side
  ADC_CLASS1_BL1 : rti1202lib_adc_class1/ADC_CLASS1_BL1  DSProperties=struct('RTI',struct('Version',uint32(1),'BlockType',struct('isSLSource',uint8(1),'isSLSink',uint8(1),'isHWSource',uint8(0),'isHWSink',uint8(1),'isSetup',uint8(0),'isInline',uint8(1),'isNonInline',uint8(0),'isInterrupt',uint8(0),'isChannelwise',uint8(1)),'IOBoardType',{{'DS120X','STD','ADCC1'}},'UnitType','ADC','Identifier','ADC','DialogType','ML','BlockSet','NONE','SlaveProcessor','NONE'))  RTIBlockInterface=struct('InputPortsActive',0,'InputPortsWidth',int32(1),'InputPortsDataType',{{'SS_BOOLEAN'}},'InputPortsName',{{'Continue'}},'OutputPortsActive',[1 0],'OutputPortsWidth',int32([1 1]),'OutputPortsDataType',{{'SS_DOUBLE','SS_INT16'}},'OutputPortsName',{{'ADC','Status'}},'DialogFcn','rti120xstdadcc1adcgui','SampleTime',{{-1}},'InitLevel',3,'IconTransparency','on','BlockDisplay',{{['ADC CL1\nChannel: 3'],'center'}},'BlockName',struct('Token',{{'ADC_CLASS1_BL1'}}))  RTIBlockParameters=struct('ReadMode',{{1,'OFF',[1 2]}},'ChannelNo',{{3,'OFF',[]}},'ConversionMode',{{1,'OFF',[1 2]}},'TriggerSource',{{1,'OFF',[1 2]}},'TriggerLineIn',{{1,'OFF',[1 16]}},'SampleMode',{{1,'OFF',[1 2]}},'BurstTriggerSource',{{1,'OFF',[1 2]}},'BurstTriggerLine',{{1,'OFF',[1 16]}},'ConvTriggerSource',{{3,'OFF',[1 3]}},'ConvTriggerLine',{{1,'OFF',[1 16]}},'ConvPeriod',{{'100e-6','OFF',[1e-6 1.34]}},'ConvPeriodCheck',{{0,'OFF',[]}},'BurstSize',{{'10','OFF',[]}},'BurstSizeCheck',{{0,'OFF',[]}},'DataSetOffset',{{'0','OFF',[]}},'DataSetOffsetCheck',{{0,'OFF',[]}},'DataSetLength',{{'1','OFF',[]}},'DataSetLengthCheck',{{0,'OFF',[]}},'EnableTriggerEvent',{{0,'OFF',[0 1]}},'TriggerMode',{{2,'OFF',[1 3]}},'TriggerLineOut',{{1,'OFF',[1 16]}},'ADCSWStartEnable',{{0,'OFF',[0 1]}},'SampleTime',{{'-1','OFF',[-1 inf]}},'SampleTimeCheck',{{1,'OFF',[]}},'StatusPortEnable',{{0,'OFF',[0 1]}},'TLCFileName',{{'rti120xadc_c1_adc','OFF',[]}})  RTISFcnParameters=struct('ReadMode','int16','ChannelNo','int16','ConversionMode','int16','TriggerSource','int16','TriggerLineIn','int16','SampleMode','int16','BurstTriggerSource','int16','BurstTriggerLine','int16','ConvTriggerSource','int16','ConvTriggerLine','int16','ConvPeriod','double','BurstSize','int16','DataSetOffset','int16','DataSetLength','int16','EnableTriggerEvent','int16','TriggerMode','int16','TriggerLineOut','int16','ADCSWStartEnable','int16','SampleTime','double','StatusPortEnable','int16','TLCFileName','char')  RTIBlockParaDefault=struct('ReadMode',1,'ChannelNo',1,'ConversionMode',1,'TriggerSource',1,'TriggerLineIn',1,'SampleMode',1,'BurstTriggerSource',1,'BurstTriggerLine',1,'ConvTriggerSource',3,'ConvTriggerLine',1,'ConvPeriod',0.0001,'ConvPeriodCheck',0,'BurstSize',10,'BurstSizeCheck',0,'DataSetOffset',0,'DataSetOffsetCheck',0,'DataSetLength',1,'DataSetLengthCheck',0,'EnableTriggerEvent',0,'TriggerMode',2,'TriggerLineOut',1,'ADCSWStartEnable',0,'SampleTime',-1,'SampleTimeCheck',1,'StatusPortEnable',0,'TLCFileName','rti120xadc_c1_adc')
  ADC_CLASS1_BL2 : rti1202lib_adc_class1/ADC_CLASS1_BL1  DSProperties=struct('RTI',struct('Version',uint32(1),'BlockType',struct('isSLSource',uint8(1),'isSLSink',uint8(1),'isHWSource',uint8(0),'isHWSink',uint8(1),'isSetup',uint8(0),'isInline',uint8(1),'isNonInline',uint8(0),'isInterrupt',uint8(0),'isChannelwise',uint8(1)),'IOBoardType',{{'DS120X','STD','ADCC1'}},'UnitType','ADC','Identifier','ADC','DialogType','ML','BlockSet','NONE','SlaveProcessor','NONE'))  RTIBlockInterface=struct('InputPortsActive',0,'InputPortsWidth',int32(1),'InputPortsDataType',{{'SS_BOOLEAN'}},'InputPortsName',{{'Continue'}},'OutputPortsActive',[1 0],'OutputPortsWidth',int32([1 1]),'OutputPortsDataType',{{'SS_DOUBLE','SS_INT16'}},'OutputPortsName',{{'ADC','Status'}},'DialogFcn','rti120xstdadcc1adcgui','SampleTime',{{-1}},'InitLevel',3,'IconTransparency','on','BlockDisplay',{{['ADC CL1\nChannel: 1'],'center'}},'BlockName',struct('Token',{{'ADC_CLASS1_BL1'}}))  RTIBlockParameters=struct('ReadMode',{{1,'OFF',[1 2]}},'ChannelNo',{{1,'OFF',[]}},'ConversionMode',{{1,'OFF',[1 2]}},'TriggerSource',{{1,'OFF',[1 2]}},'TriggerLineIn',{{1,'OFF',[1 16]}},'SampleMode',{{1,'OFF',[1 2]}},'BurstTriggerSource',{{1,'OFF',[1 2]}},'BurstTriggerLine',{{1,'OFF',[1 16]}},'ConvTriggerSource',{{3,'OFF',[1 3]}},'ConvTriggerLine',{{1,'OFF',[1 16]}},'ConvPeriod',{{'100e-6','OFF',[1e-6 1.34]}},'ConvPeriodCheck',{{0,'OFF',[]}},'BurstSize',{{'10','OFF',[]}},'BurstSizeCheck',{{0,'OFF',[]}},'DataSetOffset',{{'0','OFF',[]}},'DataSetOffsetCheck',{{0,'OFF',[]}},'DataSetLength',{{'1','OFF',[]}},'DataSetLengthCheck',{{0,'OFF',[]}},'EnableTriggerEvent',{{0,'OFF',[0 1]}},'TriggerMode',{{2,'OFF',[1 3]}},'TriggerLineOut',{{1,'OFF',[1 16]}},'ADCSWStartEnable',{{0,'OFF',[0 1]}},'SampleTime',{{'-1','OFF',[-1 inf]}},'SampleTimeCheck',{{1,'OFF',[]}},'StatusPortEnable',{{0,'OFF',[0 1]}},'TLCFileName',{{'rti120xadc_c1_adc','OFF',[]}})  RTISFcnParameters=struct('ReadMode','int16','ChannelNo','int16','ConversionMode','int16','TriggerSource','int16','TriggerLineIn','int16','SampleMode','int16','BurstTriggerSource','int16','BurstTriggerLine','int16','ConvTriggerSource','int16','ConvTriggerLine','int16','ConvPeriod','double','BurstSize','int16','DataSetOffset','int16','DataSetLength','int16','EnableTriggerEvent','int16','TriggerMode','int16','TriggerLineOut','int16','ADCSWStartEnable','int16','SampleTime','double','StatusPortEnable','int16','TLCFileName','char')  RTIBlockParaDefault=struct('ReadMode',1,'ChannelNo',1,'ConversionMode',1,'TriggerSource',1,'TriggerLineIn',1,'SampleMode',1,'BurstTriggerSource',1,'BurstTriggerLine',1,'ConvTriggerSource',3,'ConvTriggerLine',1,'ConvPeriod',0.0001,'ConvPeriodCheck',0,'BurstSize',10,'BurstSizeCheck',0,'DataSetOffset',0,'DataSetOffsetCheck',0,'DataSetLength',1,'DataSetLengthCheck',0,'EnableTriggerEvent',0,'TriggerMode',2,'TriggerLineOut',1,'ADCSWStartEnable',0,'SampleTime',-1,'SampleTimeCheck',1,'StatusPortEnable',0,'TLCFileName','rti120xadc_c1_adc')
  ADC_CLASS1_BL3 : rti1202lib_adc_class1/ADC_CLASS1_BL1  DSProperties=struct('RTI',struct('Version',uint32(1),'BlockType',struct('isSLSource',uint8(1),'isSLSink',uint8(1),'isHWSource',uint8(0),'isHWSink',uint8(1),'isSetup',uint8(0),'isInline',uint8(1),'isNonInline',uint8(0),'isInterrupt',uint8(0),'isChannelwise',uint8(1)),'IOBoardType',{{'DS120X','STD','ADCC1'}},'UnitType','ADC','Identifier','ADC','DialogType','ML','BlockSet','NONE','SlaveProcessor','NONE'))  RTIBlockInterface=struct('InputPortsActive',0,'InputPortsWidth',int32(1),'InputPortsDataType',{{'SS_BOOLEAN'}},'InputPortsName',{{'Continue'}},'OutputPortsActive',[1 0],'OutputPortsWidth',int32([1 1]),'OutputPortsDataType',{{'SS_DOUBLE','SS_INT16'}},'OutputPortsName',{{'ADC','Status'}},'DialogFcn','rti120xstdadcc1adcgui','SampleTime',{{-1}},'InitLevel',3,'IconTransparency','on','BlockDisplay',{{['ADC CL1\nChannel: 2'],'center'}},'BlockName',struct('Token',{{'ADC_CLASS1_BL1'}}))  RTIBlockParameters=struct('ReadMode',{{1,'OFF',[1 2]}},'ChannelNo',{{2,'OFF',[]}},'ConversionMode',{{1,'OFF',[1 2]}},'TriggerSource',{{1,'OFF',[1 2]}},'TriggerLineIn',{{1,'OFF',[1 16]}},'SampleMode',{{1,'OFF',[1 2]}},'BurstTriggerSource',{{1,'OFF',[1 2]}},'BurstTriggerLine',{{1,'OFF',[1 16]}},'ConvTriggerSource',{{3,'OFF',[1 3]}},'ConvTriggerLine',{{1,'OFF',[1 16]}},'ConvPeriod',{{'100e-6','OFF',[1e-6 1.34]}},'ConvPeriodCheck',{{0,'OFF',[]}},'BurstSize',{{'10','OFF',[]}},'BurstSizeCheck',{{0,'OFF',[]}},'DataSetOffset',{{'0','OFF',[]}},'DataSetOffsetCheck',{{0,'OFF',[]}},'DataSetLength',{{'1','OFF',[]}},'DataSetLengthCheck',{{0,'OFF',[]}},'EnableTriggerEvent',{{0,'OFF',[0 1]}},'TriggerMode',{{2,'OFF',[1 3]}},'TriggerLineOut',{{1,'OFF',[1 16]}},'ADCSWStartEnable',{{0,'OFF',[0 1]}},'SampleTime',{{'-1','OFF',[-1 inf]}},'SampleTimeCheck',{{1,'OFF',[]}},'StatusPortEnable',{{0,'OFF',[0 1]}},'TLCFileName',{{'rti120xadc_c1_adc','OFF',[]}})  RTISFcnParameters=struct('ReadMode','int16','ChannelNo','int16','ConversionMode','int16','TriggerSource','int16','TriggerLineIn','int16','SampleMode','int16','BurstTriggerSource','int16','BurstTriggerLine','int16','ConvTriggerSource','int16','ConvTriggerLine','int16','ConvPeriod','double','BurstSize','int16','DataSetOffset','int16','DataSetLength','int16','EnableTriggerEvent','int16','TriggerMode','int16','TriggerLineOut','int16','ADCSWStartEnable','int16','SampleTime','double','StatusPortEnable','int16','TLCFileName','char')  RTIBlockParaDefault=struct('ReadMode',1,'ChannelNo',1,'ConversionMode',1,'TriggerSource',1,'TriggerLineIn',1,'SampleMode',1,'BurstTriggerSource',1,'BurstTriggerLine',1,'ConvTriggerSource',3,'ConvTriggerLine',1,'ConvPeriod',0.0001,'ConvPeriodCheck',0,'BurstSize',10,'BurstSizeCheck',0,'DataSetOffset',0,'DataSetOffsetCheck',0,'DataSetLength',1,'DataSetLengthCheck',0,'EnableTriggerEvent',0,'TriggerMode',2,'TriggerLineOut',1,'ADCSWStartEnable',0,'SampleTime',-1,'SampleTimeCheck',1,'StatusPortEnable',0,'TLCFileName','rti120xadc_c1_adc')
  Add1 : Sum
  Divide : Product  Inputs=*/
  Divide1 : Product  Inputs=*/
  Divide2 : Product  Inputs=*/
  acc_sns1 : Gain  Gain=1000/10.2
  amp1 : Constant
  amp2 : Constant
  amp3 : Constant
  bias : Constant  Value=0
  disp_sns2 : Gain  Gain=7
  force_sns1 : Gain  Gain=1000/22.4
  in_gain1 : Gain  Gain=10
  in_gain2 : Gain  Gain=10
  in_gain3 : Gain  Gain=10
  m2mm : Gain  Gain=1000
  Out1 : Outport
  Out2 : Outport  Port=2
  Out3 : Outport  Port=3
  wires:
  ADC_CLASS1_BL2/1 -> in_gain1/1
  Divide1/1 -> disp_sns2/1
  amp2/1 -> Divide1/2
  ADC_CLASS1_BL1/1 -> in_gain2/1
  in_gain2/1 -> Divide1/1
  in_gain1/1 -> Divide/1
  Divide/1 -> force_sns1/1
  amp1/1 -> Divide/2
  force_sns1/1 -> Out1/1
  acc_sns1/1 -> m2mm/1
  amp3/1 -> Divide2/2
  ADC_CLASS1_BL3/1 -> in_gain3/1
  Divide2/1 -> acc_sns1/1
  disp_sns2/1 -> Out2/1
  m2mm/1 -> Out3/1
  in_gain3/1 -> Add1/1
  Add1/1 -> Divide2/1
  bias/1 -> Add1/2

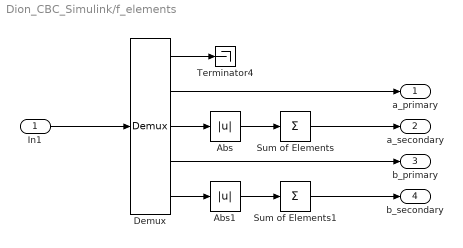
== system Dion_CBC_Simulink/f_elements ==
  In1 : Inport
  Abs : Abs  SaturateOnIntegerOverflow=off
  Abs1 : Abs  SaturateOnIntegerOverflow=off
  Demux : Demux  Outputs=[1, 1, k_harmonics-1, 1, k_harmonics-1]
  Sum of Elements : Sum  Inputs=+
  Sum of Elements1 : Sum  Inputs=+
  Terminator4 : Terminator
  a_primary : Outport
  a_secondary : Outport  Port=2
  b_primary : Outport  Port=3
  b_secondary : Outport  Port=4
  wires:
  Abs/1 -> Sum of Elements/1
  Demux/3 -> Abs/1
  Demux/1 -> Terminator4/1
  Demux/2 -> a_primary/1
  Demux/5 -> Abs1/1
  In1/1 -> Demux/1
  Abs1/1 -> Sum of Elements1/1
  Sum of Elements/1 -> a_secondary/1
  Sum of Elements1/1 -> b_secondary/1
  Demux/4 -> b_primary/1

== system Dion_CBC_Simulink/force_reconstructor ==
  coeffs : Inport
  fund_freq : Inport  Port=2
  Harmonic Basis Gen1 : Subsystem
  Product : Product
  Sum of Elements : Sum  Inputs=+
  Out1 : Outport
  wires:
  Product/1 -> Sum of Elements/1
  fund_freq/1 -> Harmonic Basis Gen1/1(fund_freq)
  Harmonic Basis Gen1/1(harmonic_basis) -> Product/2
  coeffs/1 -> Product/1
  Sum of Elements/1 -> Out1/1

== system Dion_CBC_Simulink/invasiveness_estimator ==
  x : Inport
  Abs1 : Abs  SaturateOnIntegerOverflow=off
  Abs2 : Abs  SaturateOnIntegerOverflow=off
  Divide1 : Product  Inputs=*/
  Sum of Elements : Sum  Inputs=+
  Sum of Elements1 : Sum  Inputs=+
  get primary1 : Subsystem
  get secondary : Subsystem
  invasiveness : Outport
  wires:
  get secondary/1(secondary) -> Abs1/1
  x/1 -> get secondary/1(Vector), get primary1/1(Vector)
  get primary1/1(Primary) -> Abs2/1
  Abs1/1 -> Sum of Elements/1
  Abs2/1 -> Sum of Elements1/1
  Sum of Elements/1 -> Divide1/1
  Sum of Elements1/1 -> Divide1/2
  Divide1/1 -> invasiveness/1

== system Dion_CBC_Simulink/mat2sim ==
  2D : Inport
  DC : Constant  Value=0
  Mux : Mux  Inputs=2
  Reshape : Reshape  OutputDimensionality=Customize  OutputDimensions=[2*k_harmonics,1]
  1D : Outport
  wires:
  2D/1 -> Reshape/1
  DC/1 -> Mux/1
  Mux/1 -> 1D/1
  Reshape/1 -> Mux/2

== system Dion_CBC_Simulink/sig_reconstructor ==
  coeffs : Inport
  fund_freq : Inport  Port=2
  Harmonic Basis Gen1 : Subsystem
  Product : Product
  Sum of Elements : Sum  Inputs=+
  Out1 : Outport
  wires:
  Sum of Elements/1 -> Out1/1
  coeffs/1 -> Product/1
  Harmonic Basis Gen1/1(harmonic_basis) -> Product/2
  fund_freq/1 -> Harmonic Basis Gen1/1(fund_freq)
  Product/1 -> Sum of Elements/1

== system Dion_CBC_Simulink/sim2mat ==
  1D : Inport
  Demux1 : Demux  Outputs=[1, k_harmonics, k_harmonics]
  Mux : Mux  Inputs=2
  Reshape : Reshape  OutputDimensionality=Customize  OutputDimensions=[k_harmonics,2]
  Terminator : Terminator
  2D : Outport
  wires:
  Mux/1 -> Reshape/1
  Reshape/1 -> 2D/1
  Demux1/3 -> Mux/2
  Demux1/2 -> Mux/1
  Demux1/1 -> Terminator/1
  1D/1 -> Demux1/1

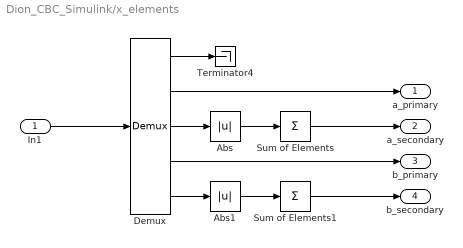
== system Dion_CBC_Simulink/x_elements ==
  In1 : Inport
  Abs : Abs  SaturateOnIntegerOverflow=off
  Abs1 : Abs  SaturateOnIntegerOverflow=off
  Demux : Demux  Outputs=[1, 1, k_harmonics-1, 1, k_harmonics-1]
  Sum of Elements : Sum  Inputs=+
  Sum of Elements1 : Sum  Inputs=+
  Terminator4 : Terminator
  a_primary : Outport
  a_secondary : Outport  Port=2
  b_primary : Outport  Port=3
  b_secondary : Outport  Port=4
  wires:
  Demux/4 -> b_primary/1
  Sum of Elements1/1 -> b_secondary/1
  Sum of Elements/1 -> a_secondary/1
  Abs1/1 -> Sum of Elements1/1
  In1/1 -> Demux/1
  Demux/5 -> Abs1/1
  Demux/2 -> a_primary/1
  Demux/1 -> Terminator4/1
  Demux/3 -> Abs/1
  Abs/1 -> Sum of Elements/1

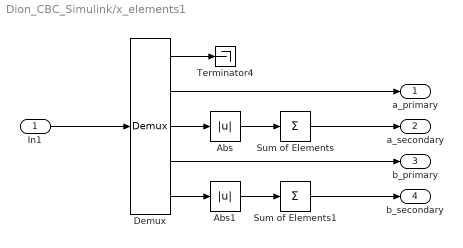
== system Dion_CBC_Simulink/x_elements1 ==
  In1 : Inport
  Abs : Abs  SaturateOnIntegerOverflow=off
  Abs1 : Abs  SaturateOnIntegerOverflow=off
  Demux : Demux  Outputs=[1, 1, k_harmonics-1, 1, k_harmonics-1]
  Sum of Elements : Sum  Inputs=+
  Sum of Elements1 : Sum  Inputs=+
  Terminator4 : Terminator
  a_primary : Outport
  a_secondary : Outport  Port=2
  b_primary : Outport  Port=3
  b_secondary : Outport  Port=4
  wires:
  Abs/1 -> Sum of Elements/1
  Demux/3 -> Abs/1
  Demux/1 -> Terminator4/1
  Demux/2 -> a_primary/1
  Demux/5 -> Abs1/1
  In1/1 -> Demux/1
  Abs1/1 -> Sum of Elements1/1
  Sum of Elements/1 -> a_secondary/1
  Sum of Elements1/1 -> b_secondary/1
  Demux/4 -> b_primary/1

== system Dion_CBC_Simulink/x_reconstructor ==
  coeffs : Inport
  fund_freq : Inport  Port=2
  Harmonic Basis Gen1 : Subsystem
  Product : Product
  Sum of Elements : Sum  Inputs=+
  Out1 : Outport
  wires:
  Sum of Elements/1 -> Out1/1
  coeffs/1 -> Product/1
  Harmonic Basis Gen1/1(harmonic_basis) -> Product/2
  fund_freq/1 -> Harmonic Basis Gen1/1(fund_freq)
  Product/1 -> Sum of Elements/1

== system Dion_CBC_Simulink/RTF_estimator/Subsystem ==
  input signal : Inport
  fund_freq : Inport  Port=2
  Fourier Series 2 : Subsystem
  Harmonic Basis Gen1 : Subsystem
  Fourier1 : Outport
  Phase1 : Outport  Port=2
  wires:
  Fourier Series 2/2(Phase) -> Phase1/1
  input signal/1 -> Fourier Series 2/1(input signal)
  Fourier Series 2/1(Fourier) -> Fourier1/1
  fund_freq/1 -> Harmonic Basis Gen1/1(fund_freq), Fourier Series 2/3(fundamental frequency)
  Harmonic Basis Gen1/1(harmonic_basis) -> Fourier Series 2/2(harmonic basis)

== system Dion_CBC_Simulink/RTF_estimator_force/Subsystem ==
  input signal : Inport
  fund_freq : Inport  Port=2
  Fourier Series 2 : Subsystem
  Harmonic Basis Gen1 : Subsystem
  Fourier1 : Outport
  Phase1 : Outport  Port=2
  wires:
  Harmonic Basis Gen1/1(harmonic_basis) -> Fourier Series 2/2(harmonic basis)
  fund_freq/1 -> Fourier Series 2/3(fundamental frequency), Harmonic Basis Gen1/1(fund_freq)
  Fourier Series 2/1(Fourier) -> Fourier1/1
  input signal/1 -> Fourier Series 2/1(input signal)
  Fourier Series 2/2(Phase) -> Phase1/1

== system Dion_CBC_Simulink/RTF_estimator_sig/Subsystem ==
  input signal : Inport
  fund_freq : Inport  Port=2
  Fourier Series 2 : Subsystem
  Harmonic Basis Gen1 : Subsystem
  Fourier1 : Outport
  Phase1 : Outport  Port=2
  wires:
  Fourier Series 2/2(Phase) -> Phase1/1
  input signal/1 -> Fourier Series 2/1(input signal)
  Fourier Series 2/1(Fourier) -> Fourier1/1
  fund_freq/1 -> Harmonic Basis Gen1/1(fund_freq), Fourier Series 2/3(fundamental frequency)
  Harmonic Basis Gen1/1(harmonic_basis) -> Fourier Series 2/2(harmonic basis)

== system Dion_CBC_Simulink/RTI Data/RTI Data Store ==
  RTI Data Store : Subsystem  mask(RTI_DATA_STORE){}
      mask help:
      | RTI Data Store Block. This block is used by RTI to store internal model dependent data. Deleting this block will result in data loss.
      |
      | NEVER DELETE, COPY, OR MODIFY THIS BLOCK!
      mask Help:
      | RTI Data Store Block. This block is used by RTI to store internal model dependent data. Deleting this block will result in data loss.
      | 
      | NEVER DELETE, COPY, OR MODIFY THIS BLOCK!
      mask Display: text(0.5, 0.5, ' ', 'HorizontalAlignment', 'center');

== system Dion_CBC_Simulink/Safety Lockout/input_safety ==
  signal : Inport
  threshold : Inport  Port=2
  Abs : Abs  SaturateOnIntegerOverflow=off
  Less Than : RelationalOperator  Operator=<  OutDataTypeStr=boolean  RndMeth=Simplest  InputSameDT=off
  valid : Outport
  wires:
  Abs/1 -> Less Than/1
  signal/1 -> Abs/1
  threshold/1 -> Less Than/2
  Less Than/1 -> valid/1

== system Dion_CBC_Simulink/Safety Lockout/output_safety ==
  signal : Inport
  threshold : Inport  Port=2
  Abs : Abs  SaturateOnIntegerOverflow=off
  Less Than : RelationalOperator  Operator=<  OutDataTypeStr=boolean  RndMeth=Simplest  InputSameDT=off
  valid : Outport
  wires:
  Less Than/1 -> valid/1
  threshold/1 -> Less Than/2
  signal/1 -> Abs/1
  Abs/1 -> Less Than/1

== system Dion_CBC_Simulink/Transience_Estimator/get primary1 ==
  Vector : Inport
  Demux : Demux  Outputs=[1, 1, k_harmonics-1, 1, k_harmonics-1]
  Mux : Mux  Inputs=2
  Terminator2 : Terminator
  Terminator3 : Terminator
  Terminator4 : Terminator
  Primary : Outport
  wires:
  Vector/1 -> Demux/1
  Demux/5 -> Terminator4/1
  Demux/3 -> Terminator3/1
  Mux/1 -> Primary/1
  Demux/4 -> Mux/2
  Demux/2 -> Mux/1
  Demux/1 -> Terminator2/1

== system Dion_CBC_Simulink/Transience_Estimator/get primary4 ==
  Vector : Inport
  Demux : Demux  Outputs=[1, 1, k_harmonics-1, 1, k_harmonics-1]
  Mux : Mux  Inputs=2
  Terminator2 : Terminator
  Terminator3 : Terminator
  Terminator4 : Terminator
  Primary : Outport
  wires:
  Demux/1 -> Terminator2/1
  Demux/2 -> Mux/1
  Demux/4 -> Mux/2
  Mux/1 -> Primary/1
  Demux/3 -> Terminator3/1
  Demux/5 -> Terminator4/1
  Vector/1 -> Demux/1

== system Dion_CBC_Simulink/Transience_Estimator_force/get primary1 ==
  Vector : Inport
  Demux : Demux  Outputs=[1, 1, k_harmonics-1, 1, k_harmonics-1]
  Mux : Mux  Inputs=2
  Terminator2 : Terminator
  Terminator3 : Terminator
  Terminator4 : Terminator
  Primary : Outport
  wires:
  Demux/1 -> Terminator2/1
  Demux/2 -> Mux/1
  Demux/4 -> Mux/2
  Mux/1 -> Primary/1
  Demux/3 -> Terminator3/1
  Demux/5 -> Terminator4/1
  Vector/1 -> Demux/1

== system Dion_CBC_Simulink/Transience_Estimator_force/get primary4 ==
  Vector : Inport
  Demux : Demux  Outputs=[1, 1, k_harmonics-1, 1, k_harmonics-1]
  Mux : Mux  Inputs=2
  Terminator2 : Terminator
  Terminator3 : Terminator
  Terminator4 : Terminator
  Primary : Outport
  wires:
  Vector/1 -> Demux/1
  Demux/5 -> Terminator4/1
  Demux/3 -> Terminator3/1
  Mux/1 -> Primary/1
  Demux/4 -> Mux/2
  Demux/2 -> Mux/1
  Demux/1 -> Terminator2/1

== system Dion_CBC_Simulink/Transience_Estimator_sig/get primary1 ==
  Vector : Inport
  Demux : Demux  Outputs=[1, 1, k_harmonics-1, 1, k_harmonics-1]
  Mux : Mux  Inputs=2
  Terminator2 : Terminator
  Terminator3 : Terminator
  Terminator4 : Terminator
  Primary : Outport
  wires:
  Vector/1 -> Demux/1
  Demux/5 -> Terminator4/1
  Demux/3 -> Terminator3/1
  Mux/1 -> Primary/1
  Demux/4 -> Mux/2
  Demux/2 -> Mux/1
  Demux/1 -> Terminator2/1

== system Dion_CBC_Simulink/Transience_Estimator_sig/get primary4 ==
  Vector : Inport
  Demux : Demux  Outputs=[1, 1, k_harmonics-1, 1, k_harmonics-1]
  Mux : Mux  Inputs=2
  Terminator2 : Terminator
  Terminator3 : Terminator
  Terminator4 : Terminator
  Primary : Outport
  wires:
  Demux/1 -> Terminator2/1
  Demux/2 -> Mux/1
  Demux/4 -> Mux/2
  Mux/1 -> Primary/1
  Demux/3 -> Terminator3/1
  Demux/5 -> Terminator4/1
  Vector/1 -> Demux/1

== system Dion_CBC_Simulink/force_reconstructor/Harmonic Basis Gen1 ==
  fund_freq : Inport
  Cos : Trigonometry  Operator=cos
  DC : Constant
  Gain1 : Gain  Gain=2*pi
  Integrator : Integrator
  Mux : Mux  Inputs=3
  Product : Product
  Sin : Trigonometry
  harmonics_array : Constant  Value=1:k_harmonics
  harmonic_basis : Outport  OutDataTypeStr=double  SampleTime=0
  wires:
  DC/1 -> Mux/1
  fund_freq/1 -> Integrator/1
  harmonics_array/1 -> Product/2
  Sin/1 -> Mux/3
  Product/1 -> Gain1/1
  Cos/1 -> Mux/2
  Integrator/1 -> Product/1
  Mux/1 -> harmonic_basis/1
  Gain1/1 -> Cos/1, Sin/1

== system Dion_CBC_Simulink/invasiveness_estimator/get primary1 ==
  Vector : Inport
  Demux : Demux  Outputs=[1, 1, k_harmonics-1, 1, k_harmonics-1]
  Mux : Mux  Inputs=2
  Terminator2 : Terminator
  Terminator3 : Terminator
  Terminator4 : Terminator
  Primary : Outport
  wires:
  Vector/1 -> Demux/1
  Demux/5 -> Terminator4/1
  Demux/3 -> Terminator3/1
  Mux/1 -> Primary/1
  Demux/4 -> Mux/2
  Demux/2 -> Mux/1
  Demux/1 -> Terminator2/1
